simulink model "lookup_nD_TestGen27"  (R2017b)
settings: Solver=FixedStepDiscrete  StartTime=0.0  StopTime=10.0  RelTol=1e-3
model workspace (MAT data in the model file):
  LUTObjLKnD27 = Simulink.LookupTable
  LUTObjLKnD27.Table = Simulink.lookuptable.Table
  LUTObjLKnD27.Table.Value = reshape([4 16 10 4 16 10 4 16 10 4 16 10 4 16 10 4 16 10 5 19 18 5 19 18 5 19 18 5 19 18 5 19 18 5 19 18 6 20 23 6 20 23 6 20 23 6 20 23 6 20 23 6 20 23 7 21 24 7 21 24 7 21 24 7 21 24 7 21 24 7 21 24 8 22 25 8 22 25 8 22 25 8 22 25 8 22 25 8 22 25 4 16 10 4 16 10 4 16 10 4 16 10 4 16 10 4 16 10 5 19 18 5 19 18 5 19 18 5 19 18 5 19 18 5 19 18 6 20 23 6 20 23 6 20 23 6 20 23 6 20 23 6 20 23 7 21 24 7 21 24 7 21 24 7 21 24 7 21 24 7 21 24 8 22 25 8 22 25 8 22 25 8 22 25 8 22 25 8 22 25], [2 5 3 2 3])
  LUTObjLKnD27.Table.Dimensions = [2 5 3 2 3]
  LUTObjLKnD27.Table.DataType = 'double'
  LUTObjLKnD27.Table.FieldName = 'Table'
  LUTObjLKnD27.Breakpoints(1) = Simulink.lookuptable.Breakpoint
  LUTObjLKnD27.Breakpoints(1).Value = [39.1443760763; 108.28152529]
  LUTObjLKnD27.Breakpoints(1).TunableSizeName = 'N1'
  LUTObjLKnD27.Breakpoints(1).Dimensions = [2 1]
  LUTObjLKnD27.Breakpoints(1).DataType = 'double'
  LUTObjLKnD27.Breakpoints(1).FieldName = 'BP1'
  LUTObjLKnD27.Breakpoints(2) = Simulink.lookuptable.Breakpoint
  LUTObjLKnD27.Breakpoints(2).Value = [41.7378793693; 58.210446971; 103.319508928; 115.383023816; 125.893322999]
  LUTObjLKnD27.Breakpoints(2).TunableSizeName = 'N2'
  LUTObjLKnD27.Breakpoints(2).Dimensions = [5 1]
  LUTObjLKnD27.Breakpoints(2).DataType = 'double'
  LUTObjLKnD27.Breakpoints(2).FieldName = 'BP2'
  LUTObjLKnD27.Breakpoints(3) = Simulink.lookuptable.Breakpoint
  LUTObjLKnD27.Breakpoints(3).Value = [37.4727238815; 40.2478273813; 111.237234779]
  LUTObjLKnD27.Breakpoints(3).TunableSizeName = 'N3'
  LUTObjLKnD27.Breakpoints(3).Dimensions = [3 1]
  LUTObjLKnD27.Breakpoints(3).DataType = 'double'
  LUTObjLKnD27.Breakpoints(3).FieldName = 'BP3'
  LUTObjLKnD27.Breakpoints(4) = Simulink.lookuptable.Breakpoint
  LUTObjLKnD27.Breakpoints(4).Value = [117.931540575; 121.892353448]
  LUTObjLKnD27.Breakpoints(4).TunableSizeName = 'N4'
  LUTObjLKnD27.Breakpoints(4).Dimensions = [2 1]
  LUTObjLKnD27.Breakpoints(4).DataType = 'double'
  LUTObjLKnD27.Breakpoints(4).FieldName = 'BP4'
  LUTObjLKnD27.Breakpoints(5) = Simulink.lookuptable.Breakpoint
  LUTObjLKnD27.Breakpoints(5).Value = [62.4534779611; 63.0097457613; 126.010029592]
  LUTObjLKnD27.Breakpoints(5).TunableSizeName = 'N5'
  LUTObjLKnD27.Breakpoints(5).Dimensions = [3 1]
  LUTObjLKnD27.Breakpoints(5).DataType = 'double'
  LUTObjLKnD27.Breakpoints(5).FieldName = 'BP5'
  LUTObjLKnD27.SupportTunableSize = 0
  LUTObjLKnD27.StructTypeInfo = Simulink.lookuptable.StructTypeInfo
  LUTObjLKnD27.StructTypeInfo.Name = 'LUT'
  LUTObjLKnD27.StructTypeInfo.DataScope = 'Auto'
settings Model: Creator=ktrinh  LastModifiedBy=ktrinh
settings DebuggingCC: ParameterOverflowMsg=none

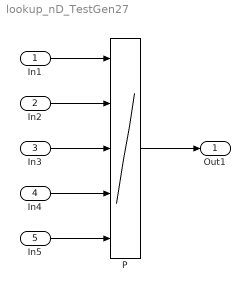
== system lookup_nD_TestGen27 ==
  In1 : Inport  OutMin=0  OutMax=127  PortDimensions=[2,3]
  In2 : Inport  Port=2  OutMin=0  OutMax=127
  In3 : Inport  Port=3  OutMin=0  OutMax=127
  In4 : Inport  Port=4  OutMin=0  OutMax=127
  In5 : Inport  Port=5  OutMin=0  OutMax=127
  P : Lookup_n-D  NumberOfTableDimensions=5  DataSpecification=Lookup table object  LookupTableObject=LUTObjLKnD27  BreakpointsForDimension3=[5, 7]  Table=reshape(repmat([4 5 6;16 19 20;10 18 23],1,2),[3,3,2])  InterpMethod=Nearest  ExtrapMethod=Clip  UseLastTableValue=on  InternalRulePriority=Speed  OutDataTypeStr=double  RndMeth=Zero  SaturateOnIntegerOverflow=on  InputSameDT=on
  Out1 : Outport
  wires:
  In1/1 -> P/1
  In2/1 -> P/2
  In3/1 -> P/3
  In4/1 -> P/4
  In5/1 -> P/5
  P/1 -> Out1/1
